simulink library "Crazyflie_Library"  (R2019a)
settings: Solver=VariableStepAuto  StartTime=0.0  StopTime=10.0  RelTol=1e-3
values from neighbouring files (symbols this model uses):
  DeePC_param = evalin('base', 'DeePC_param')    [DeePC_Optimizer_osqp.m]
  param = evalin('base', 'param')    [DeePC_Optimizer_osqp.m]    (also in DeePC_main.m = load_crazyflie_parameters(i_aux))
undefined symbols (not defined in the file or in its folder): DiscIntNeverNeededParam
libraries: simulink x3, $bdroot x3
(part 1 of 2)
settings Model: Creator=ezzat  LastModifiedBy=ezzat
settings DataIOCC: ReturnWorkspaceOutputs=off
settings DebuggingCC: ArithmeticOperatorsInVariantConditions=warning

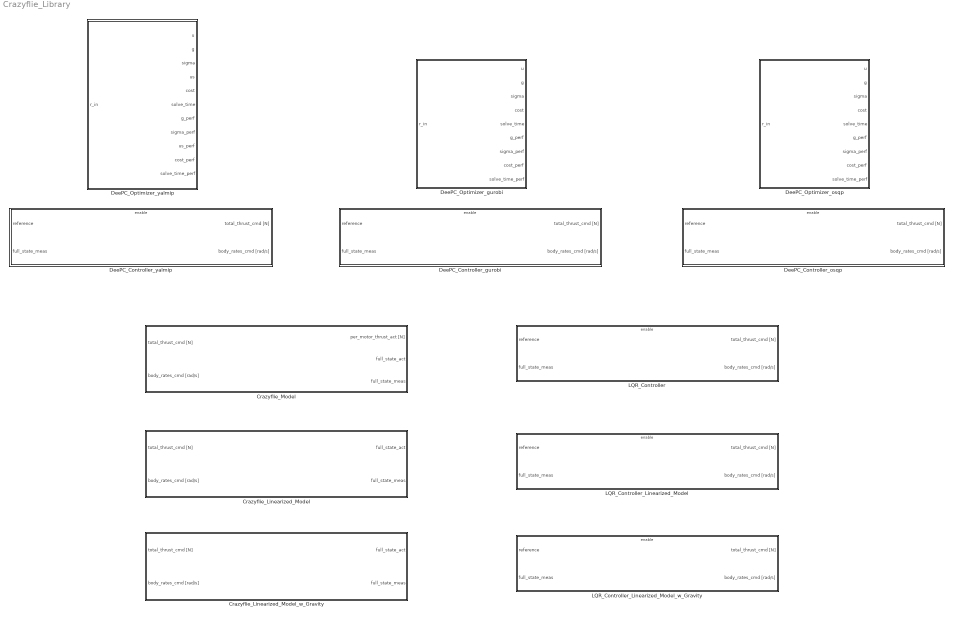
== system Crazyflie_Library ==
  Crazyflie_Linearized_Model : Subsystem
  Crazyflie_Linearized_Model_w_Gravity : Subsystem
  Crazyflie_Model : Subsystem
  DeePC_Controller_gurobi : Subsystem
  DeePC_Controller_osqp : Subsystem
  DeePC_Controller_yalmip : Subsystem
  DeePC_Optimizer_gurobi : Subsystem
  DeePC_Optimizer_osqp : Subsystem
  DeePC_Optimizer_yalmip : Subsystem
  LQR_Controller : Subsystem
  LQR_Controller_Linearized_Model : Subsystem
  LQR_Controller_Linearized_Model_w_Gravity : Subsystem

== system Crazyflie_Library/Crazyflie_Linearized_Model ==
  note: full state measurement
      | (x, y, z, x_dot, y_dot, z_dot, roll, pitch, yaw, roll_dot, pitch_dot, yaw_dot)
  total_thrust_cmd [N] : Inport
  body_rates_cmd [rad/s] : Inport  Port=2
  Add : Sum
  Gain : Gain  Gain=param.Bc  Multiplication=Matrix(K*u)
  Gain1 : Gain  Gain=param.Ac  Multiplication=Matrix(K*u)
  Integrator : Integrator  InitialCondition=param.nrotor_initial_condition(1:9)
  Measurements : Subsystem
  Mux : Mux  Inputs=2
  Mux1 : Mux  Inputs=2
  Unit Delay : UnitDelay  InitialCondition=param.nrotor_initial_condition(10:12)  SampleTime=param.sample_time_controller_inner  HasFrameUpgradeWarning=on
  full_state_act : Outport
  full_state_meas : Outport  Port=2
  wires:
  Measurements/1(full state measurements) -> full_state_meas/1
  total_thrust_cmd [N]/1 -> Mux/1
  body_rates_cmd [rad/s]/1 -> Unit Delay/1, Mux/2
  Mux/1 -> Gain/1
  Gain/1 -> Add/1
  Gain1/1 -> Add/2
  Add/1 -> Integrator/1
  Integrator/1 -> Mux1/1, Gain1/1
  Mux1/1 -> full_state_act/1, Measurements/1(full state)
  Unit Delay/1 -> Mux1/2

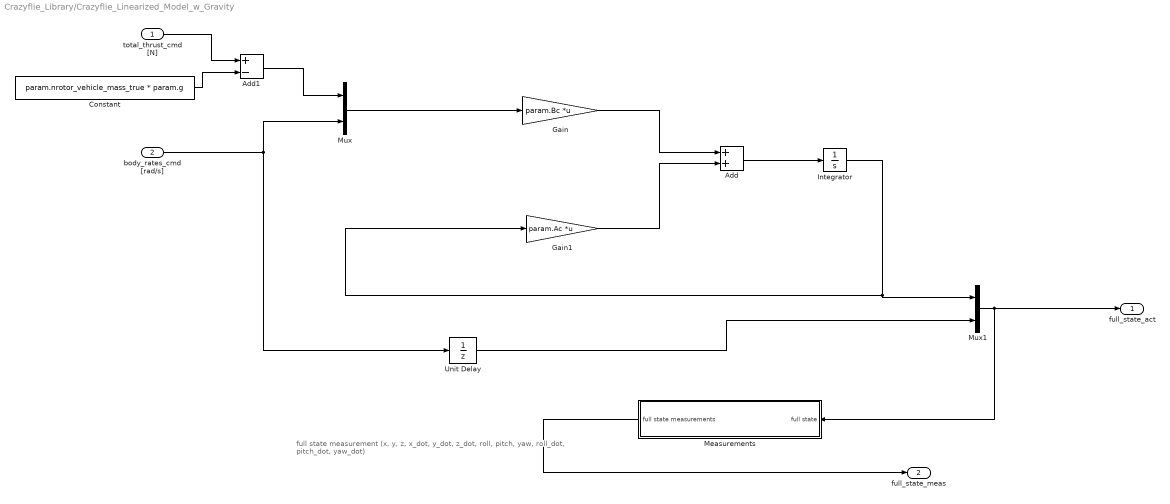
== system Crazyflie_Library/Crazyflie_Linearized_Model_w_Gravity ==
  note: full state measurement
      | (x, y, z, x_dot, y_dot, z_dot, roll, pitch, yaw, roll_dot, pitch_dot, yaw_dot)
  total_thrust_cmd [N] : Inport
  body_rates_cmd [rad/s] : Inport  Port=2
  Add : Sum
  Add1 : Sum  Inputs=+-
  Constant : Constant  Value=param.nrotor_vehicle_mass_true * param.g
  Gain : Gain  Gain=param.Bc  Multiplication=Matrix(K*u)
  Gain1 : Gain  Gain=param.Ac  Multiplication=Matrix(K*u)
  Integrator : Integrator  InitialCondition=param.nrotor_initial_condition(1:9)
  Measurements : Subsystem
  Mux : Mux  Inputs=2
  Mux1 : Mux  Inputs=2
  Unit Delay : UnitDelay  InitialCondition=param.nrotor_initial_condition(10:12)  SampleTime=param.sample_time_controller_inner  HasFrameUpgradeWarning=on
  full_state_act : Outport
  full_state_meas : Outport  Port=2
  wires:
  Measurements/1(full state measurements) -> full_state_meas/1
  body_rates_cmd [rad/s]/1 -> Unit Delay/1, Mux/2
  Mux/1 -> Gain/1
  Gain/1 -> Add/1
  Gain1/1 -> Add/2
  Add/1 -> Integrator/1
  Integrator/1 -> Mux1/1, Gain1/1
  Mux1/1 -> full_state_act/1, Measurements/1(full state)
  total_thrust_cmd [N]/1 -> Add1/1
  Add1/1 -> Mux/1
  Constant/1 -> Add1/2
  Unit Delay/1 -> Mux1/2

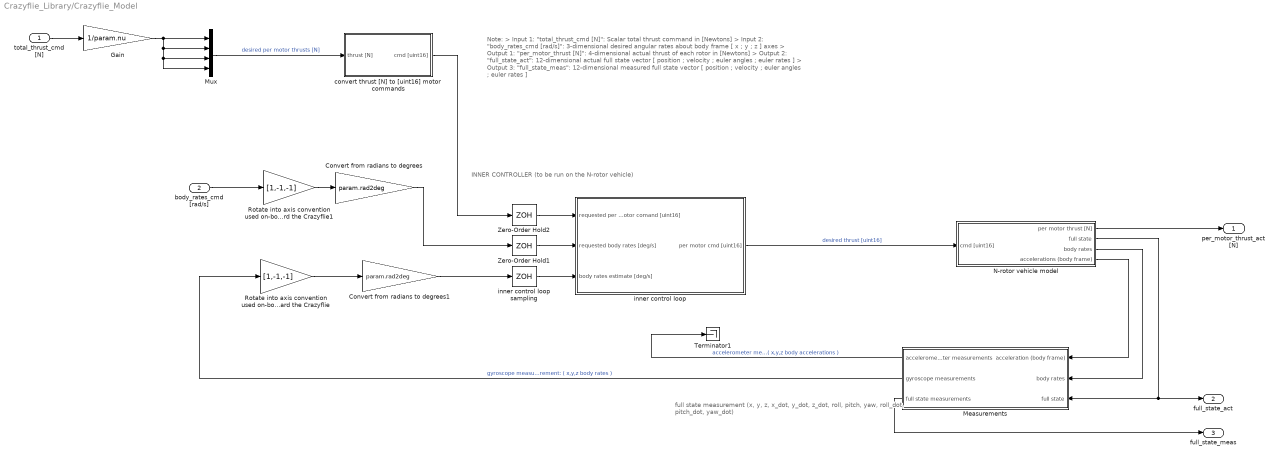
== system Crazyflie_Library/Crazyflie_Model ==
  note: Note:
      | > Input 1: "total_thrust_cmd [N]": Scalar total thrust command in [Newtons]
      | > Input 2: "body_rates_cmd [rad/s]": 3-dimensional desired angular rates about body frame [ x ; y ; z ] axes
      | > Output 1: "per_motor_thrust [N]": 4-dimensional actual thrust of each rotor in [Newtons]
      | > Output 2: "full_state_act": 12-dimensional actual full state vector [ position ; velocity ; euler angles ; euler rates ]
      | > Output 3: "full_state_meas": 12-dimensional measured full state vector [ position ; velocity ; euler angles ; euler rates ]
  note: full state measurement
      | (x, y, z, x_dot, y_dot, z_dot, roll, pitch, yaw, roll_dot, pitch_dot, yaw_dot)
  note: INNER CONTROLLER (to be run on the N-rotor vehicle)
  total_thrust_cmd [N] : Inport
  body_rates_cmd [rad/s] : Inport  Port=2
  Convert from radians to degrees : Gain  Gain=param.rad2deg
  Convert from radians to degrees1 : Gain  Gain=param.rad2deg
  Gain : Gain  Gain=1/param.nu
  Measurements : Subsystem
  Mux : Mux  Inputs=param.nu
  N-rotor vehicle model : Subsystem
  Rotate into axis convention used on-board the Crazyflie1 : Gain  Gain=[1,-1,-1]
  Rotate into axis convention used on-board the Crazyflie : Gain  Gain=[1,-1,-1]
  Terminator1 : Terminator
  Zero-Order Hold1 : ZeroOrderHold  SampleTime=param.sample_time_controller_inner
  Zero-Order Hold2 : ZeroOrderHold  SampleTime=param.sample_time_controller_inner
  convert thrust [N] to [uint16] motor commands : Subsystem
  inner control loop sampling : ZeroOrderHold  SampleTime=param.sample_time_controller_inner
  inner control loop : Subsystem
  "per_motor_thrust_act [N] " : Outport
  full_state_act : Outport  Port=2
  full_state_meas : Outport  Port=3
  wires:
  Gain/1 -> Mux/4, Mux/3, Mux/2, Mux/1
  Zero-Order Hold1/1 -> inner control loop/2(requested body rates [deg/s])
  Convert from radians to degrees/1 -> Zero-Order Hold1/1
  Mux/1 -> convert thrust [N] to [uint16] motor commands/1(thrust [N])  "desired per motor thrusts [N]"
  Measurements/1(accelerometer measurements) -> Terminator1/1  "accelerometer measurement: ( x,y,z body accelerations )"
  N-rotor vehicle model/2(full state) -> Measurements/3(full state), full_state_act/1
  body_rates_cmd [rad/s]/1 -> Rotate into axis convention used on-board the Crazyflie1/1
  N-rotor vehicle model/1(per motor thrust [N]) -> "per_motor_thrust_act [N] "/1
  N-rotor vehicle model/3(body rates) -> Measurements/2(body rates)
  Measurements/3(full state measurements) -> full_state_meas/1
  Convert from radians to degrees1/1 -> inner control loop sampling/1
  inner control loop/1(per motor cmd [uint16]) -> N-rotor vehicle model/1(cmd [uint16])  "desired thrust [uint16]"
  Rotate into axis convention used on-board the Crazyflie/1 -> Convert from radians to degrees1/1
  Zero-Order Hold2/1 -> inner control loop/1(requested per motor comand [uint16])
  N-rotor vehicle model/4(accelerations (body frame)) -> Measurements/1(acceleration (body frame))
  total_thrust_cmd [N]/1 -> Gain/1
  convert thrust [N] to [uint16] motor commands/1(cmd [uint16]) -> Zero-Order Hold2/1
  inner control loop sampling/1 -> inner control loop/3(body rates estimate [deg/s])
  Measurements/2(gyroscope measurements) -> Rotate into axis convention used on-board the Crazyflie/1  "gyroscope measurement: ( x,y,z body rates )"
  Rotate into axis convention used on-board the Crazyflie1/1 -> Convert from radians to degrees/1

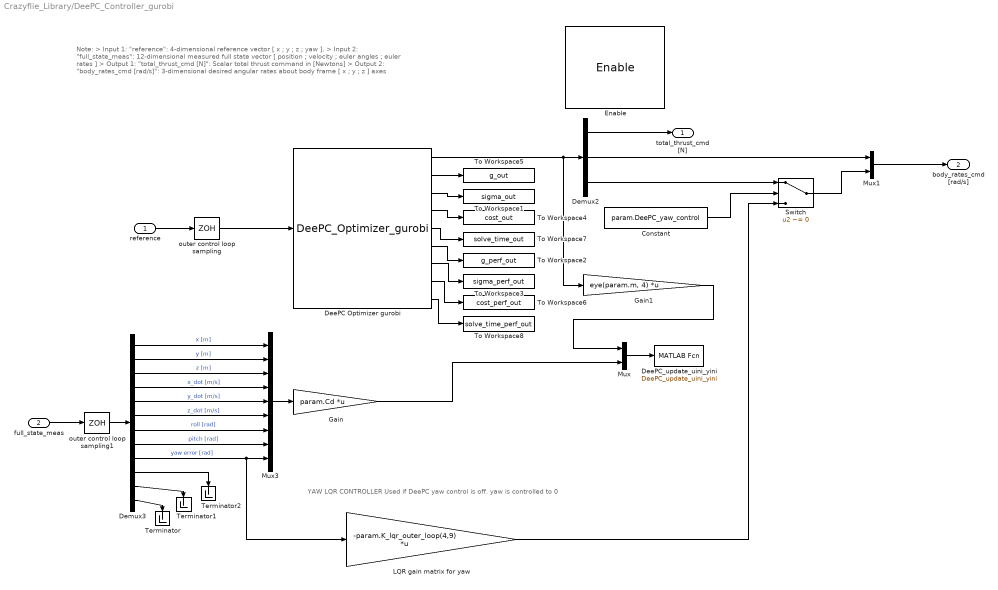
== system Crazyflie_Library/DeePC_Controller_gurobi ==
  note: Note:
      | > Input 1: "reference": 4-dimensional reference vector [ x ; y ; z ; yaw ].
      | > Input 2: "full_state_meas": 12-dimensional measured full state vector [ position ; velocity ; euler angles ; euler rates ]
      | > Output 1: "total_thrust_cmd [N]": Scalar total thrust command in [Newtons]
      | > Output 2: "body_rates_cmd [rad/s]": 3-dimensional desired angular rates about body frame [ x ; y ; z ] axes
  note: YAW LQR CONTROLLER
      | Used if DeePC yaw control is off. yaw is controlled to 0
  reference : Inport
  full_state_meas : Inport  Port=2
  Enable : EnablePort
  Constant : Constant  Value=param.DeePC_yaw_control
  DeePC Optimizer gurobi : $bdroot/DeePC_Optimizer_gurobi  SystemSampleTime=-1
  DeePC_update_uini_yini : MATLABFcn  MATLABFcn=DeePC_update_uini_yini  OutputDimensions=0
  Demux2 : Demux  Outputs=[1 2 1]
  Demux3 : Demux  Outputs=12
  Gain : Gain  Gain=param.Cd  Multiplication=Matrix(K*u)
  Gain1 : Gain  Gain=eye(param.m, 4)  Multiplication=Matrix(K*u)
  LQR gain matrix for yaw : Gain  Gain=-param.K_lqr_outer_loop(4,9)  Multiplication=Matrix(K*u)
  Mux : Mux  Inputs=2
  Mux1 : Mux  Inputs=[2 1]
  Mux3 : Mux  Inputs=9
  Switch : Switch  Criteria=u2 ~= 0
  Terminator : Terminator
  Terminator1 : Terminator
  Terminator2 : Terminator
  To Workspace1 : ToWorkspace  VariableName=sigma_out  SampleTime=-1
  To Workspace2 : ToWorkspace  VariableName=g_perf_out  SampleTime=-1
  To Workspace3 : ToWorkspace  VariableName=sigma_perf_out  SampleTime=-1
  To Workspace4 : ToWorkspace  VariableName=cost_out  SampleTime=-1
  To Workspace5 : ToWorkspace  VariableName=g_out  SampleTime=-1
  To Workspace6 : ToWorkspace  VariableName=cost_perf_out  SampleTime=-1
  To Workspace7 : ToWorkspace  VariableName=solve_time_out  SampleTime=-1
  To Workspace8 : ToWorkspace  VariableName=solve_time_perf_out  SampleTime=-1
  outer control loop sampling : ZeroOrderHold  SampleTime=param.sample_time_controller_outer
  outer control loop sampling1 : ZeroOrderHold  SampleTime=param.sample_time_controller_outer
  total_thrust_cmd [N] : Outport
  body_rates_cmd [rad/s] : Outport  Port=2
  wires:
  Demux3/11 -> Terminator1/1
  Demux3/1 -> Mux3/1  "x [m]"
  Demux3/3 -> Mux3/3  "z [m]"
  Demux3/6 -> Mux3/6  "z_dot [m/s]"
  Demux3/2 -> Mux3/2  "y [m]"
  Demux3/8 -> Mux3/8  "pitch [rad]"
  Demux3/12 -> Terminator/1
  Demux3/7 -> Mux3/7  "roll [rad]"
  Demux3/10 -> Terminator2/1
  Demux3/4 -> Mux3/4  "x_dot [m/s]"
  Demux3/5 -> Mux3/5  "y_dot [m/s]"
  full_state_meas/1 -> outer control loop sampling1/1
  reference/1 -> outer control loop sampling/1
  outer control loop sampling1/1 -> Demux3/1
  Mux3/1 -> Gain/1
  Demux2/1 -> total_thrust_cmd [N]/1
  outer control loop sampling/1 -> DeePC Optimizer gurobi/1
  Mux/1 -> DeePC_update_uini_yini/1
  Gain/1 -> Mux/2
  DeePC Optimizer gurobi/1 -> Gain1/1, Demux2/1
  Demux2/2 -> Mux1/1
  Mux1/1 -> body_rates_cmd [rad/s]/1
  LQR gain matrix for yaw/1 -> Switch/3
  Demux3/9 -> LQR gain matrix for yaw/1, Mux3/9  "yaw error [rad]"
  Demux2/3 -> Switch/1
  Switch/1 -> Mux1/2
  Constant/1 -> Switch/2
  Gain1/1 -> Mux/1
  DeePC Optimizer gurobi/2 -> To Workspace5/1
  DeePC Optimizer gurobi/9 -> To Workspace8/1
  DeePC Optimizer gurobi/5 -> To Workspace7/1
  DeePC Optimizer gurobi/6 -> To Workspace2/1
  DeePC Optimizer gurobi/8 -> To Workspace6/1
  DeePC Optimizer gurobi/3 -> To Workspace1/1
  DeePC Optimizer gurobi/4 -> To Workspace4/1
  DeePC Optimizer gurobi/7 -> To Workspace3/1

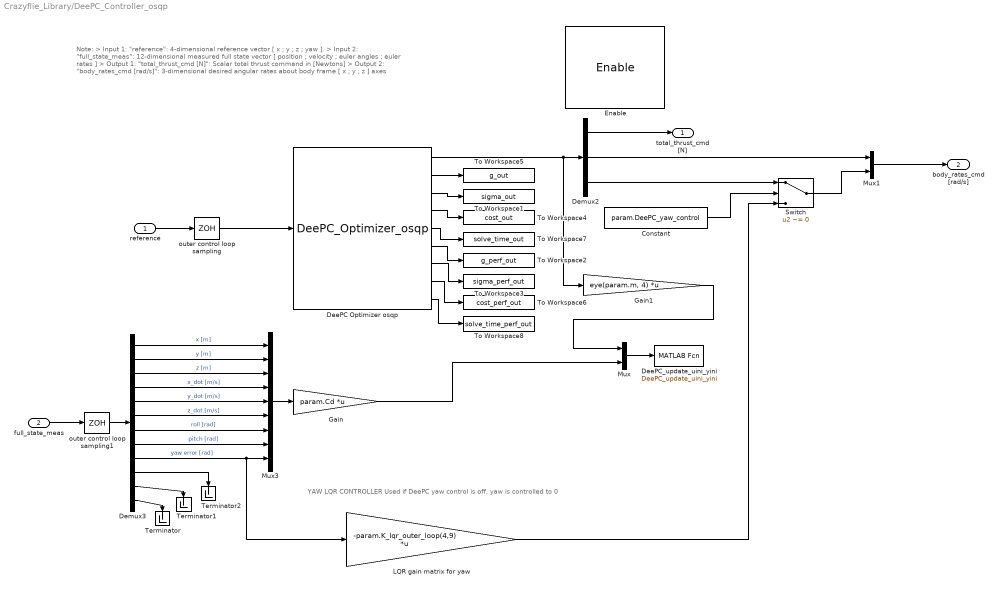
== system Crazyflie_Library/DeePC_Controller_osqp ==
  note: Note:
      | > Input 1: "reference": 4-dimensional reference vector [ x ; y ; z ; yaw ].
      | > Input 2: "full_state_meas": 12-dimensional measured full state vector [ position ; velocity ; euler angles ; euler rates ]
      | > Output 1: "total_thrust_cmd [N]": Scalar total thrust command in [Newtons]
      | > Output 2: "body_rates_cmd [rad/s]": 3-dimensional desired angular rates about body frame [ x ; y ; z ] axes
  note: YAW LQR CONTROLLER
      | Used if DeePC yaw control is off. yaw is controlled to 0
  reference : Inport
  full_state_meas : Inport  Port=2
  Enable : EnablePort
  Constant : Constant  Value=param.DeePC_yaw_control
  DeePC Optimizer osqp : $bdroot/DeePC_Optimizer_osqp  SystemSampleTime=-1
  DeePC_update_uini_yini : MATLABFcn  MATLABFcn=DeePC_update_uini_yini  OutputDimensions=0
  Demux2 : Demux  Outputs=[1 2 1]
  Demux3 : Demux  Outputs=12
  Gain : Gain  Gain=param.Cd  Multiplication=Matrix(K*u)
  Gain1 : Gain  Gain=eye(param.m, 4)  Multiplication=Matrix(K*u)
  LQR gain matrix for yaw : Gain  Gain=-param.K_lqr_outer_loop(4,9)  Multiplication=Matrix(K*u)
  Mux : Mux  Inputs=2
  Mux1 : Mux  Inputs=[2 1]
  Mux3 : Mux  Inputs=9
  Switch : Switch  Criteria=u2 ~= 0
  Terminator : Terminator
  Terminator1 : Terminator
  Terminator2 : Terminator
  To Workspace1 : ToWorkspace  VariableName=sigma_out  SampleTime=-1
  To Workspace2 : ToWorkspace  VariableName=g_perf_out  SampleTime=-1
  To Workspace3 : ToWorkspace  VariableName=sigma_perf_out  SampleTime=-1
  To Workspace4 : ToWorkspace  VariableName=cost_out  SampleTime=-1
  To Workspace5 : ToWorkspace  VariableName=g_out  SampleTime=-1
  To Workspace6 : ToWorkspace  VariableName=cost_perf_out  SampleTime=-1
  To Workspace7 : ToWorkspace  VariableName=solve_time_out  SampleTime=-1
  To Workspace8 : ToWorkspace  VariableName=solve_time_perf_out  SampleTime=-1
  outer control loop sampling : ZeroOrderHold  SampleTime=param.sample_time_controller_outer
  outer control loop sampling1 : ZeroOrderHold  SampleTime=param.sample_time_controller_outer
  total_thrust_cmd [N] : Outport
  body_rates_cmd [rad/s] : Outport  Port=2
  wires:
  Demux3/11 -> Terminator1/1
  Demux3/1 -> Mux3/1  "x [m]"
  Demux3/3 -> Mux3/3  "z [m]"
  Demux3/6 -> Mux3/6  "z_dot [m/s]"
  Demux3/2 -> Mux3/2  "y [m]"
  Demux3/8 -> Mux3/8  "pitch [rad]"
  Demux3/12 -> Terminator/1
  Demux3/7 -> Mux3/7  "roll [rad]"
  Demux3/10 -> Terminator2/1
  Demux3/4 -> Mux3/4  "x_dot [m/s]"
  Demux3/5 -> Mux3/5  "y_dot [m/s]"
  full_state_meas/1 -> outer control loop sampling1/1
  reference/1 -> outer control loop sampling/1
  outer control loop sampling1/1 -> Demux3/1
  Mux3/1 -> Gain/1
  Demux2/1 -> total_thrust_cmd [N]/1
  outer control loop sampling/1 -> DeePC Optimizer osqp/1
  Mux/1 -> DeePC_update_uini_yini/1
  Gain/1 -> Mux/2
  DeePC Optimizer osqp/1 -> Gain1/1, Demux2/1
  Demux2/2 -> Mux1/1
  Mux1/1 -> body_rates_cmd [rad/s]/1
  LQR gain matrix for yaw/1 -> Switch/3
  Demux3/9 -> LQR gain matrix for yaw/1, Mux3/9  "yaw error [rad]"
  Demux2/3 -> Switch/1
  Switch/1 -> Mux1/2
  Constant/1 -> Switch/2
  Gain1/1 -> Mux/1
  DeePC Optimizer osqp/2 -> To Workspace5/1
  DeePC Optimizer osqp/9 -> To Workspace8/1
  DeePC Optimizer osqp/5 -> To Workspace7/1
  DeePC Optimizer osqp/6 -> To Workspace2/1
  DeePC Optimizer osqp/8 -> To Workspace6/1
  DeePC Optimizer osqp/3 -> To Workspace1/1
  DeePC Optimizer osqp/4 -> To Workspace4/1
  DeePC Optimizer osqp/7 -> To Workspace3/1

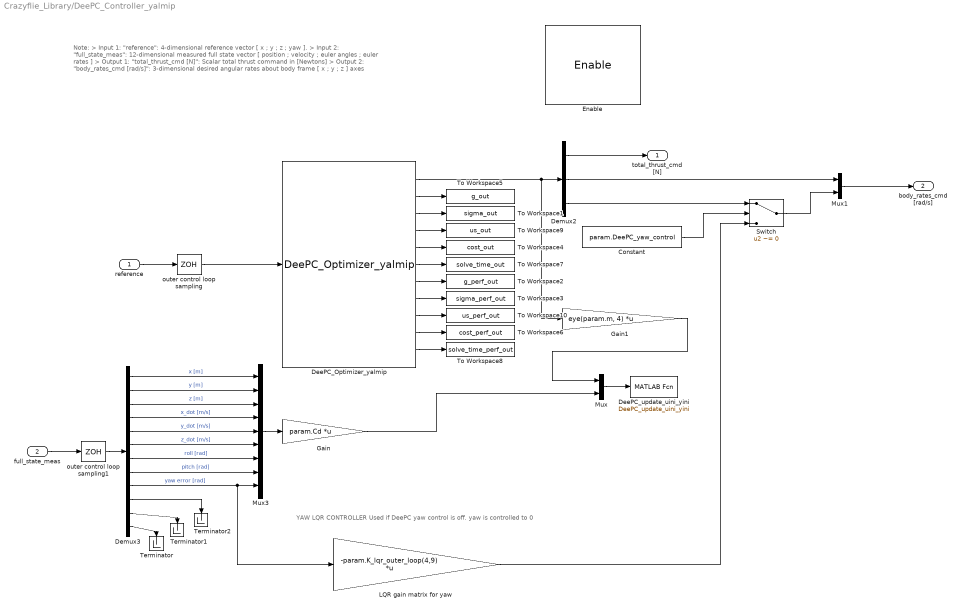
== system Crazyflie_Library/DeePC_Controller_yalmip ==
  note: Note:
      | > Input 1: "reference": 4-dimensional reference vector [ x ; y ; z ; yaw ].
      | > Input 2: "full_state_meas": 12-dimensional measured full state vector [ position ; velocity ; euler angles ; euler rates ]
      | > Output 1: "total_thrust_cmd [N]": Scalar total thrust command in [Newtons]
      | > Output 2: "body_rates_cmd [rad/s]": 3-dimensional desired angular rates about body frame [ x ; y ; z ] axes
  note: YAW LQR CONTROLLER
      | Used if DeePC yaw control is off. yaw is controlled to 0
  reference : Inport
  full_state_meas : Inport  Port=2
  Enable : EnablePort
  Constant : Constant  Value=param.DeePC_yaw_control
  DeePC_Optimizer_yalmip : $bdroot/DeePC_Optimizer_yalmip  SystemSampleTime=-1
  DeePC_update_uini_yini : MATLABFcn  MATLABFcn=DeePC_update_uini_yini  OutputDimensions=0
  Demux2 : Demux  Outputs=[1 2 1]
  Demux3 : Demux  Outputs=12
  Gain : Gain  Gain=param.Cd  Multiplication=Matrix(K*u)
  Gain1 : Gain  Gain=eye(param.m, 4)  Multiplication=Matrix(K*u)
  LQR gain matrix for yaw : Gain  Gain=-param.K_lqr_outer_loop(4,9)  Multiplication=Matrix(K*u)
  Mux : Mux  Inputs=2
  Mux1 : Mux  Inputs=[2 1]
  Mux3 : Mux  Inputs=9
  Switch : Switch  Criteria=u2 ~= 0
  Terminator : Terminator
  Terminator1 : Terminator
  Terminator2 : Terminator
  To Workspace1 : ToWorkspace  VariableName=sigma_out  SampleTime=-1
  To Workspace10 : ToWorkspace  VariableName=us_perf_out  SampleTime=-1
  To Workspace2 : ToWorkspace  VariableName=g_perf_out  SampleTime=-1
  To Workspace3 : ToWorkspace  VariableName=sigma_perf_out  SampleTime=-1
  To Workspace4 : ToWorkspace  VariableName=cost_out  SampleTime=-1
  To Workspace5 : ToWorkspace  VariableName=g_out  SampleTime=-1
  To Workspace6 : ToWorkspace  VariableName=cost_perf_out  SampleTime=-1
  To Workspace7 : ToWorkspace  VariableName=solve_time_out  SampleTime=-1
  To Workspace8 : ToWorkspace  VariableName=solve_time_perf_out  SampleTime=-1
  To Workspace9 : ToWorkspace  VariableName=us_out  SampleTime=-1
  outer control loop sampling : ZeroOrderHold  SampleTime=param.sample_time_controller_outer
  outer control loop sampling1 : ZeroOrderHold  SampleTime=param.sample_time_controller_outer
  total_thrust_cmd [N] : Outport
  body_rates_cmd [rad/s] : Outport  Port=2
  wires:
  Demux3/11 -> Terminator1/1
  Demux3/1 -> Mux3/1  "x [m]"
  Demux3/3 -> Mux3/3  "z [m]"
  Demux3/6 -> Mux3/6  "z_dot [m/s]"
  Demux3/2 -> Mux3/2  "y [m]"
  Demux3/8 -> Mux3/8  "pitch [rad]"
  Demux3/12 -> Terminator/1
  Demux3/7 -> Mux3/7  "roll [rad]"
  Demux3/10 -> Terminator2/1
  Demux3/4 -> Mux3/4  "x_dot [m/s]"
  Demux3/5 -> Mux3/5  "y_dot [m/s]"
  full_state_meas/1 -> outer control loop sampling1/1
  reference/1 -> outer control loop sampling/1
  outer control loop sampling1/1 -> Demux3/1
  Mux3/1 -> Gain/1
  Demux2/1 -> total_thrust_cmd [N]/1
  DeePC_Optimizer_yalmip/2 -> To Workspace5/1
  DeePC_Optimizer_yalmip/3 -> To Workspace1/1
  outer control loop sampling/1 -> DeePC_Optimizer_yalmip/1
  Mux/1 -> DeePC_update_uini_yini/1
  Gain/1 -> Mux/2
  Demux2/2 -> Mux1/1
  Mux1/1 -> body_rates_cmd [rad/s]/1
  LQR gain matrix for yaw/1 -> Switch/3
  Demux3/9 -> LQR gain matrix for yaw/1, Mux3/9  "yaw error [rad]"
  Demux2/3 -> Switch/1
  Switch/1 -> Mux1/2
  Constant/1 -> Switch/2
  Gain1/1 -> Mux/1
  DeePC_Optimizer_yalmip/1 -> Gain1/1, Demux2/1
  DeePC_Optimizer_yalmip/5 -> To Workspace4/1
  DeePC_Optimizer_yalmip/4 -> To Workspace9/1
  DeePC_Optimizer_yalmip/6 -> To Workspace7/1
  DeePC_Optimizer_yalmip/7 -> To Workspace2/1
  DeePC_Optimizer_yalmip/8 -> To Workspace3/1
  DeePC_Optimizer_yalmip/11 -> To Workspace8/1
  DeePC_Optimizer_yalmip/10 -> To Workspace6/1
  DeePC_Optimizer_yalmip/9 -> To Workspace10/1

== system Crazyflie_Library/DeePC_Optimizer_gurobi ==
  r_in : Inport
  DeePC_Optimizer_gurobi : MATLABFcn  MATLABFcn=DeePC_Optimizer_gurobi  OutputDimensions=2 * (DeePC_param.Ng + DeePC_param.Ns + 2) + 4
  Demux : Demux  Outputs=[DeePC_param.Ng DeePC_param.Ns 1 1 DeePC_param.Ng DeePC_param.Ns 1 1 4]
  u : Outport
  g : Outport  Port=2
  sigma : Outport  Port=3
  cost : Outport  Port=4
  solve_time : Outport  Port=5
  g_perf : Outport  Port=6
  sigma_perf : Outport  Port=7
  cost_perf : Outport  Port=8
  solve_time_perf : Outport  Port=9
  wires:
  r_in/1 -> DeePC_Optimizer_gurobi/1
  Demux/8 -> solve_time_perf/1
  Demux/6 -> sigma_perf/1
  Demux/2 -> sigma/1
  Demux/4 -> solve_time/1
  Demux/9 -> u/1
  Demux/5 -> g_perf/1
  Demux/7 -> cost_perf/1
  Demux/1 -> g/1
  DeePC_Optimizer_gurobi/1 -> Demux/1
  Demux/3 -> cost/1

== system Crazyflie_Library/DeePC_Optimizer_osqp ==
  r_in : Inport
  DeePC_Optimizer_osqp : MATLABFcn  MATLABFcn=DeePC_Optimizer_osqp  OutputDimensions=2 * (DeePC_param.Ng + DeePC_param.Ns + 2) + 4
  Demux : Demux  Outputs=[DeePC_param.Ng DeePC_param.Ns 1 1 DeePC_param.Ng DeePC_param.Ns 1 1 4]
  u : Outport
  g : Outport  Port=2
  sigma : Outport  Port=3
  cost : Outport  Port=4
  solve_time : Outport  Port=5
  g_perf : Outport  Port=6
  sigma_perf : Outport  Port=7
  cost_perf : Outport  Port=8
  solve_time_perf : Outport  Port=9
  wires:
  r_in/1 -> DeePC_Optimizer_osqp/1
  Demux/8 -> solve_time_perf/1
  Demux/6 -> sigma_perf/1
  Demux/2 -> sigma/1
  Demux/4 -> solve_time/1
  Demux/9 -> u/1
  Demux/5 -> g_perf/1
  Demux/7 -> cost_perf/1
  Demux/1 -> g/1
  DeePC_Optimizer_osqp/1 -> Demux/1
  Demux/3 -> cost/1

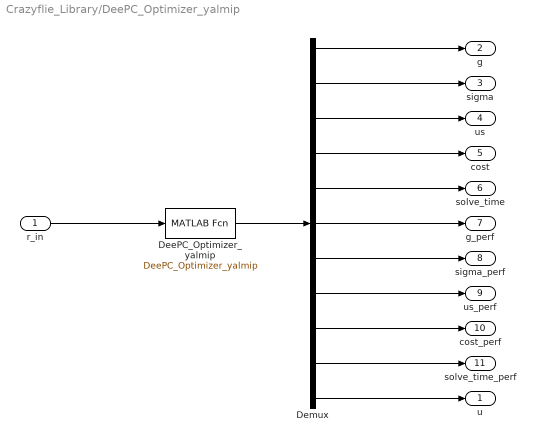
== system Crazyflie_Library/DeePC_Optimizer_yalmip ==
  r_in : Inport
  DeePC_Optimizer_yalmip : MATLABFcn  MATLABFcn=DeePC_Optimizer_yalmip  OutputDimensions=2 * (DeePC_param.Ng + DeePC_param.Ns + param.m + 2) + 4
  Demux : Demux  Outputs=[DeePC_param.Ng DeePC_param.Ns param.m 1 1 DeePC_param.Ng DeePC_param.Ns param.m 1 1 4]
  u : Outport
  g : Outport  Port=2
  sigma : Outport  Port=3
  us : Outport  Port=4
  cost : Outport  Port=5
  solve_time : Outport  Port=6
  g_perf : Outport  Port=7
  sigma_perf : Outport  Port=8
  us_perf : Outport  Port=9
  cost_perf : Outport  Port=10
  solve_time_perf : Outport  Port=11
  wires:
  DeePC_Optimizer_yalmip/1 -> Demux/1
  Demux/1 -> g/1
  Demux/2 -> sigma/1
  r_in/1 -> DeePC_Optimizer_yalmip/1
  Demux/11 -> u/1
  Demux/10 -> solve_time_perf/1
  Demux/9 -> cost_perf/1
  Demux/7 -> sigma_perf/1
  Demux/6 -> g_perf/1
  Demux/5 -> solve_time/1
  Demux/4 -> cost/1
  Demux/3 -> us/1
  Demux/8 -> us_perf/1

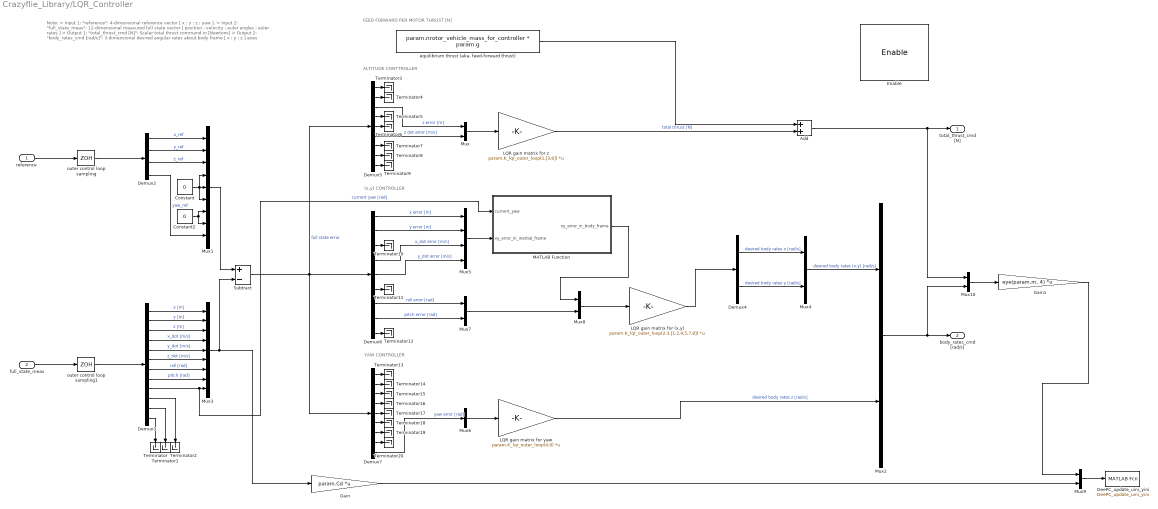
== system Crazyflie_Library/LQR_Controller ==
  note: Note:
      | > Input 1: "reference": 4-dimensional reference vector [ x ; y ; z ; yaw ].
      | > Input 2: "full_state_meas": 12-dimensional measured full state vector [ position ; velocity ; euler angles ; euler rates ]
      | > Output 1: "total_thrust_cmd [N]": Scalar total thrust command in [Newtons]
      | > Output 2: "body_rates_cmd [rad/s]": 3-dimensional desired angular rates about body frame [ x ; y ; z ] axes
  note: ALTITUDE CONTTROLLER
  note: FEED FORWARD PER MOTOR THRUST [N]
  note: YAW CONTROLLER
  note: (x,y) CONTROLLER
  reference : Inport
  full_state_meas : Inport  Port=2
  Enable : EnablePort
  Add : Sum
  Constant : Constant  Value=0
  Constant2 : Constant  Value=0
  DeePC_update_uini_yini : MATLABFcn  MATLABFcn=DeePC_update_uini_yini  OutputDimensions=0
  Demux2 : Demux
  Demux3 : Demux  Outputs=12
  Demux4 : Demux  Outputs=2
  Demux5 : Demux  Outputs=9
  Demux6 : Demux  Outputs=9
  Demux7 : Demux  Outputs=9
  Gain : Gain  Gain=param.Cd  Multiplication=Matrix(K*u)
  Gain1 : Gain  Gain=eye(param.m, 4)  Multiplication=Matrix(K*u)
  LQR gain matrix for (x,y) : Gain  Gain=param.K_lqr_outer_loop(2:3,[1,2,4,5,7,8])  Multiplication=Matrix(K*u)
  LQR gain matrix for yaw : Gain  Gain=param.K_lqr_outer_loop(4,9)  Multiplication=Matrix(K*u)
  LQR gain matrix for z : Gain  Gain=param.K_lqr_outer_loop(1,[3,6])  Multiplication=Matrix(K*u)
  MATLAB Function : MATLAB Function  TreatAsAtomicUnit=on
  Mux{,2,4,7..10} (7 alike) : Mux  Inputs=2
  Mux1 : Mux  Inputs=9
  Mux3 : Mux  Inputs=9
  Mux5 : Mux
  Mux6 : Mux  Inputs=1
  Subtract : Sum  Inputs=+-
  Terminator{,1..20} (21 alike) : Terminator
  equilibrium thrust (aka. feed-forward thrust) : Constant  Value=param.nrotor_vehicle_mass_for_controller * param.g
  outer control loop sampling : ZeroOrderHold  SampleTime=param.sample_time_controller_outer
  outer control loop sampling1 : ZeroOrderHold  SampleTime=param.sample_time_controller_outer
  total_thrust_cmd [N] : Outport
  body_rates_cmd [rad/s] : Outport  Port=2
  wires:
  outer control loop sampling1/1 -> Demux3/1
  reference/1 -> outer control loop sampling/1
  outer control loop sampling/1 -> Demux2/1
  full_state_meas/1 -> outer control loop sampling1/1
  Demux5/1 -> Terminator3/1
  Demux5/5 -> Terminator6/1
  Demux3/5 -> Mux3/5  "y_dot [m/s]"
  Demux4/1 -> Mux4/1  "desired body rates x [rad/s]"
  LQR gain matrix for (x,y)/1 -> Demux4/1
  Demux5/7 -> Terminator7/1
  Mux8/1 -> LQR gain matrix for (x,y)/1
  Mux1/1 -> Subtract/1
  Demux7/7 -> Terminator19/1
  MATLAB Function/1(xy_error_in_body_frame) -> Mux8/1
  Demux6/1 -> Mux5/1  "x error [m]"
  Demux5/2 -> Terminator4/1
  Mux6/1 -> LQR gain matrix for yaw/1
  Demux6/3 -> Terminator10/1
  Demux5/9 -> Terminator9/1
  Mux5/1 -> MATLAB Function/2(xy_error_in_inertial_frame)
  Demux7/8 -> Terminator20/1
  Demux5/3 -> Mux/1  "z error [m]"
  Demux7/1 -> Terminator13/1
  Demux6/7 -> Mux7/1  "roll error [rad]"
  Mux/1 -> LQR gain matrix for z/1
  Demux2/3 -> Mux1/3  "z_ref"
  Demux3/4 -> Mux3/4  "x_dot [m/s]"
  Demux6/8 -> Mux7/2  "pitch error [rad]"
  Demux6/2 -> Mux5/2  "y error [m]"
  Demux5/8 -> Terminator8/1
  Demux6/9 -> Terminator12/1
  Demux7/2 -> Terminator14/1
  LQR gain matrix for yaw/1 -> Mux2/2  "desired body rates z [rad/s]"
  Demux4/2 -> Mux4/2  "desired body rates y [rad/s]"
  Subtract/1 -> Demux7/1, Demux5/1, Demux6/1  "full state error"
  Demux3/10 -> Terminator2/1
  Demux5/6 -> Mux/2  "z dot error [m/s]"
  Demux2/2 -> Mux1/2  "y_ref"
  Demux3/7 -> Mux3/7  "roll [rad]"
  Demux3/9 -> MATLAB Function/1(current_yaw), Mux3/9  "current yaw [rad]"
  Demux3/12 -> Terminator/1
  Demux6/4 -> Mux5/3  "x_dot error [m/s]"
  Demux3/8 -> Mux3/8  "pitch [rad]"
  Demux2/4 -> Mux1/9  "yaw_ref"
  Demux3/2 -> Mux3/2  "y [m]"
  Demux6/6 -> Terminator11/1
  Constant2/1 -> Mux1/8, Mux1/7
  Constant/1 -> Mux1/6, Mux1/4, Mux1/5
  Demux6/5 -> Mux5/4  "y_dot error [m/s]"
  Demux3/6 -> Mux3/6  "z_dot [m/s]"
  Demux3/3 -> Mux3/3  "z [m]"
  Mux4/1 -> Mux2/1  "desired body rates (x,y) [rad/s]"
  Demux7/3 -> Terminator15/1
  Demux3/1 -> Mux3/1  "x [m]"
  Mux7/1 -> Mux8/2
  Demux2/1 -> Mux1/1  "x_ref"
  Demux7/6 -> Terminator18/1
  Demux7/5 -> Terminator17/1
  LQR gain matrix for z/1 -> Add/2  "total thrust [N]"
  Demux7/9 -> Mux6/1  "yaw error [rad]"
  Demux3/11 -> Terminator1/1
  Demux5/4 -> Terminator5/1
  Demux7/4 -> Terminator16/1
  equilibrium thrust (aka. feed-forward thrust)/1 -> Add/1
  Mux9/1 -> DeePC_update_uini_yini/1
  Add/1 -> total_thrust_cmd [N]/1, Mux10/1
  Mux2/1 -> Mux10/2, body_rates_cmd [rad/s]/1
  Mux3/1 -> Gain/1, Subtract/2
  Gain/1 -> Mux9/2
  Gain1/1 -> Mux9/1
  Mux10/1 -> Gain1/1

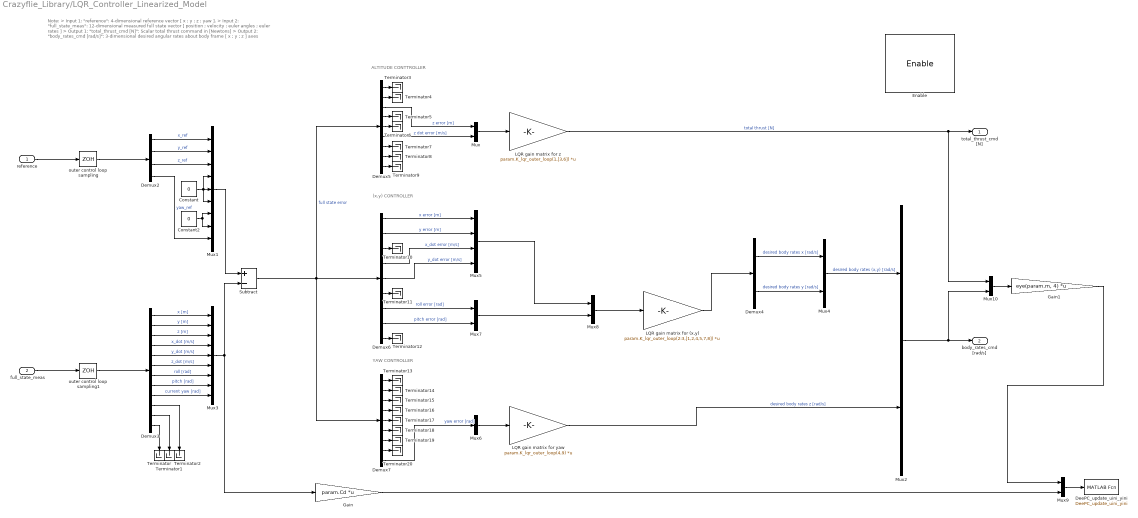
== system Crazyflie_Library/LQR_Controller_Linearized_Model ==
  note: Note:
      | > Input 1: "reference": 4-dimensional reference vector [ x ; y ; z ; yaw ].
      | > Input 2: "full_state_meas": 12-dimensional measured full state vector [ position ; velocity ; euler angles ; euler rates ]
      | > Output 1: "total_thrust_cmd [N]": Scalar total thrust command in [Newtons]
      | > Output 2: "body_rates_cmd [rad/s]": 3-dimensional desired angular rates about body frame [ x ; y ; z ] axes
  note: ALTITUDE CONTTROLLER
  note: YAW CONTROLLER
  note: (x,y) CONTROLLER
  reference : Inport
  full_state_meas : Inport  Port=2
  Enable : EnablePort
  Constant : Constant  Value=0
  Constant2 : Constant  Value=0
  DeePC_update_uini_yini : MATLABFcn  MATLABFcn=DeePC_update_uini_yini  OutputDimensions=0
  Demux2 : Demux
  Demux3 : Demux  Outputs=12
  Demux4 : Demux  Outputs=2
  Demux5 : Demux  Outputs=9
  Demux6 : Demux  Outputs=9
  Demux7 : Demux  Outputs=9
  Gain : Gain  Gain=param.Cd  Multiplication=Matrix(K*u)
  Gain1 : Gain  Gain=eye(param.m, 4)  Multiplication=Matrix(K*u)
  LQR gain matrix for (x,y) : Gain  Gain=param.K_lqr_outer_loop(2:3,[1,2,4,5,7,8])  Multiplication=Matrix(K*u)
  LQR gain matrix for yaw : Gain  Gain=param.K_lqr_outer_loop(4,9)  Multiplication=Matrix(K*u)
  LQR gain matrix for z : Gain  Gain=param.K_lqr_outer_loop(1,[3,6])  Multiplication=Matrix(K*u)
  Mux{,2,4,7..10} (7 alike) : Mux  Inputs=2
  Mux1 : Mux  Inputs=9
  Mux3 : Mux  Inputs=9
  Mux5 : Mux
  Mux6 : Mux  Inputs=1
  Subtract : Sum  Inputs=+-
  Terminator{,1..20} (21 alike) : Terminator
  outer control loop sampling : ZeroOrderHold  SampleTime=param.sample_time_controller_outer
  outer control loop sampling1 : ZeroOrderHold  SampleTime=param.sample_time_controller_outer
  total_thrust_cmd [N] : Outport
  body_rates_cmd [rad/s] : Outport  Port=2
  wires:
  outer control loop sampling1/1 -> Demux3/1
  reference/1 -> outer control loop sampling/1
  outer control loop sampling/1 -> Demux2/1
  full_state_meas/1 -> outer control loop sampling1/1
  Demux5/1 -> Terminator3/1
  Demux5/5 -> Terminator6/1
  Demux3/5 -> Mux3/5  "y_dot [m/s]"
  Demux4/1 -> Mux4/1  "desired body rates x [rad/s]"
  LQR gain matrix for (x,y)/1 -> Demux4/1
  Demux5/7 -> Terminator7/1
  Mux8/1 -> LQR gain matrix for (x,y)/1
  Mux1/1 -> Subtract/1
  Demux7/7 -> Terminator19/1
  Mux5/1 -> Mux8/1
  Demux6/1 -> Mux5/1  "x error [m]"
  Demux5/2 -> Terminator4/1
  Mux6/1 -> LQR gain matrix for yaw/1
  Demux6/3 -> Terminator10/1
  Demux5/9 -> Terminator9/1
  Demux7/8 -> Terminator20/1
  Demux5/3 -> Mux/1  "z error [m]"
  Demux7/1 -> Terminator13/1
  Demux6/7 -> Mux7/1  "roll error [rad]"
  Mux/1 -> LQR gain matrix for z/1
  Demux2/3 -> Mux1/3  "z_ref"
  Demux3/4 -> Mux3/4  "x_dot [m/s]"
  Demux6/8 -> Mux7/2  "pitch error [rad]"
  Demux6/2 -> Mux5/2  "y error [m]"
  Demux5/8 -> Terminator8/1
  Demux6/9 -> Terminator12/1
  Demux7/2 -> Terminator14/1
  LQR gain matrix for yaw/1 -> Mux2/2  "desired body rates z [rad/s]"
  Demux4/2 -> Mux4/2  "desired body rates y [rad/s]"
  Subtract/1 -> Demux7/1, Demux5/1, Demux6/1  "full state error"
  Demux3/10 -> Terminator2/1
  Demux5/6 -> Mux/2  "z dot error [m/s]"
  Demux2/2 -> Mux1/2  "y_ref"
  Demux3/7 -> Mux3/7  "roll [rad]"
  Demux3/9 -> Mux3/9  "current yaw [rad]"
  Demux3/12 -> Terminator/1
  Demux6/4 -> Mux5/3  "x_dot error [m/s]"
  Demux3/8 -> Mux3/8  "pitch [rad]"
  Demux2/4 -> Mux1/9  "yaw_ref"
  Demux3/2 -> Mux3/2  "y [m]"
  Demux6/6 -> Terminator11/1
  Constant2/1 -> Mux1/8, Mux1/7
  Constant/1 -> Mux1/6, Mux1/4, Mux1/5
  Demux6/5 -> Mux5/4  "y_dot error [m/s]"
  Demux3/6 -> Mux3/6  "z_dot [m/s]"
  Demux3/3 -> Mux3/3  "z [m]"
  Mux4/1 -> Mux2/1  "desired body rates (x,y) [rad/s]"
  Demux7/3 -> Terminator15/1
  Demux3/1 -> Mux3/1  "x [m]"
  Mux7/1 -> Mux8/2
  Demux2/1 -> Mux1/1  "x_ref"
  Demux7/6 -> Terminator18/1
  Demux7/5 -> Terminator17/1
  LQR gain matrix for z/1 -> Mux10/1, total_thrust_cmd [N]/1  "total thrust [N]"
  Demux7/9 -> Mux6/1  "yaw error [rad]"
  Demux3/11 -> Terminator1/1
  Demux5/4 -> Terminator5/1
  Demux7/4 -> Terminator16/1
  Mux9/1 -> DeePC_update_uini_yini/1
  Mux2/1 -> Mux10/2, body_rates_cmd [rad/s]/1
  Mux3/1 -> Subtract/2, Gain/1
  Gain/1 -> Mux9/2
  Mux10/1 -> Gain1/1
  Gain1/1 -> Mux9/1

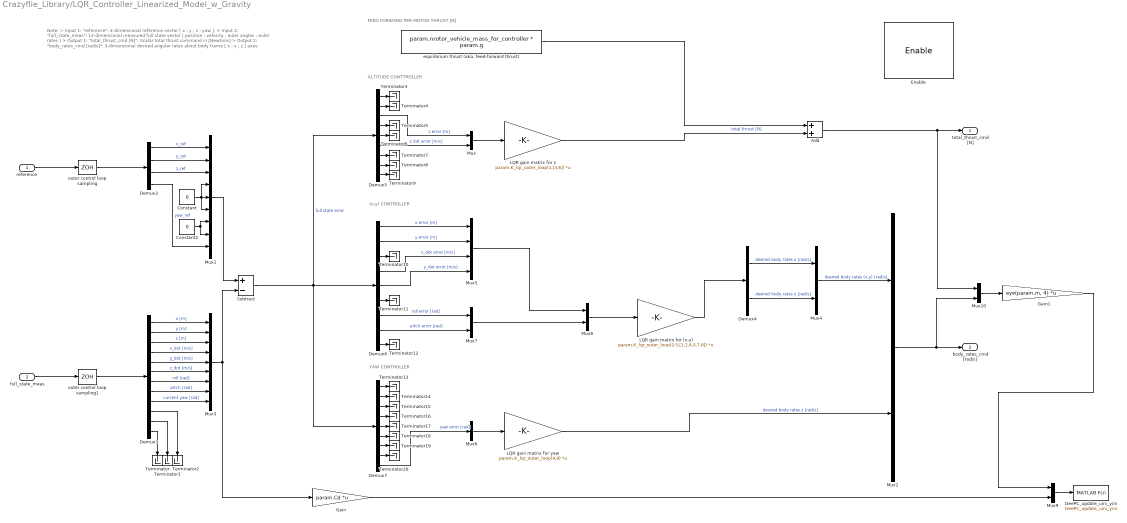
== system Crazyflie_Library/LQR_Controller_Linearized_Model_w_Gravity ==
  note: Note:
      | > Input 1: "reference": 4-dimensional reference vector [ x ; y ; z ; yaw ].
      | > Input 2: "full_state_meas": 12-dimensional measured full state vector [ position ; velocity ; euler angles ; euler rates ]
      | > Output 1: "total_thrust_cmd [N]": Scalar total thrust command in [Newtons]
      | > Output 2: "body_rates_cmd [rad/s]": 3-dimensional desired angular rates about body frame [ x ; y ; z ] axes
  note: ALTITUDE CONTTROLLER
  note: YAW CONTROLLER
  note: (x,y) CONTROLLER
  note: FEED FORWARD PER MOTOR THRUST [N]
  reference : Inport
  full_state_meas : Inport  Port=2
  Enable : EnablePort
  Add : Sum
  Constant : Constant  Value=0
  Constant2 : Constant  Value=0
  DeePC_update_uini_yini : MATLABFcn  MATLABFcn=DeePC_update_uini_yini  OutputDimensions=0
  Demux2 : Demux
  Demux3 : Demux  Outputs=12
  Demux4 : Demux  Outputs=2
  Demux5 : Demux  Outputs=9
  Demux6 : Demux  Outputs=9
  Demux7 : Demux  Outputs=9
  Gain : Gain  Gain=param.Cd  Multiplication=Matrix(K*u)
  Gain1 : Gain  Gain=eye(param.m, 4)  Multiplication=Matrix(K*u)
  LQR gain matrix for (x,y) : Gain  Gain=param.K_lqr_outer_loop(2:3,[1,2,4,5,7,8])  Multiplication=Matrix(K*u)
  LQR gain matrix for yaw : Gain  Gain=param.K_lqr_outer_loop(4,9)  Multiplication=Matrix(K*u)
  LQR gain matrix for z : Gain  Gain=param.K_lqr_outer_loop(1,[3,6])  Multiplication=Matrix(K*u)
  Mux{,2,4,7..10} (7 alike) : Mux  Inputs=2
  Mux1 : Mux  Inputs=9
  Mux3 : Mux  Inputs=9
  Mux5 : Mux
  Mux6 : Mux  Inputs=1
  Subtract : Sum  Inputs=+-
  Terminator{,1..20} (21 alike) : Terminator
  equilibrium thrust (aka. feed-forward thrust) : Constant  Value=param.nrotor_vehicle_mass_for_controller * param.g
  outer control loop sampling : ZeroOrderHold  SampleTime=param.sample_time_controller_outer
  outer control loop sampling1 : ZeroOrderHold  SampleTime=param.sample_time_controller_outer
  total_thrust_cmd [N] : Outport
  body_rates_cmd [rad/s] : Outport  Port=2
  wires:
  Mux2/1 -> Mux10/2, body_rates_cmd [rad/s]/1
  outer control loop sampling1/1 -> Demux3/1
  reference/1 -> outer control loop sampling/1
  outer control loop sampling/1 -> Demux2/1
  full_state_meas/1 -> outer control loop sampling1/1
  Demux5/1 -> Terminator3/1
  Demux5/5 -> Terminator6/1
  Demux3/5 -> Mux3/5  "y_dot [m/s]"
  Demux4/1 -> Mux4/1  "desired body rates x [rad/s]"
  LQR gain matrix for (x,y)/1 -> Demux4/1
  Demux5/7 -> Terminator7/1
  Mux8/1 -> LQR gain matrix for (x,y)/1
  Mux1/1 -> Subtract/1
  Demux7/7 -> Terminator19/1
  Mux5/1 -> Mux8/1
  Demux6/1 -> Mux5/1  "x error [m]"
  Demux5/2 -> Terminator4/1
  Mux6/1 -> LQR gain matrix for yaw/1
  Demux6/3 -> Terminator10/1
  Demux5/9 -> Terminator9/1
  Demux7/8 -> Terminator20/1
  Demux5/3 -> Mux/1  "z error [m]"
  Demux7/1 -> Terminator13/1
  Demux6/7 -> Mux7/1  "roll error [rad]"
  Mux/1 -> LQR gain matrix for z/1
  Demux2/3 -> Mux1/3  "z_ref"
  Demux3/4 -> Mux3/4  "x_dot [m/s]"
  Demux6/8 -> Mux7/2  "pitch error [rad]"
  Demux6/2 -> Mux5/2  "y error [m]"
  Demux5/8 -> Terminator8/1
  Demux6/9 -> Terminator12/1
  Demux7/2 -> Terminator14/1
  LQR gain matrix for yaw/1 -> Mux2/2  "desired body rates z [rad/s]"
  Demux4/2 -> Mux4/2  "desired body rates y [rad/s]"
  Subtract/1 -> Demux7/1, Demux5/1, Demux6/1  "full state error"
  Demux3/10 -> Terminator2/1
  Demux5/6 -> Mux/2  "z dot error [m/s]"
  Demux2/2 -> Mux1/2  "y_ref"
  Demux3/7 -> Mux3/7  "roll [rad]"
  Demux3/9 -> Mux3/9  "current yaw [rad]"
  Demux3/12 -> Terminator/1
  Demux6/4 -> Mux5/3  "x_dot error [m/s]"
  Demux3/8 -> Mux3/8  "pitch [rad]"
  Demux2/4 -> Mux1/9  "yaw_ref"
  Demux3/2 -> Mux3/2  "y [m]"
  Demux6/6 -> Terminator11/1
  Constant2/1 -> Mux1/8, Mux1/7
  Constant/1 -> Mux1/6, Mux1/4, Mux1/5
  Demux6/5 -> Mux5/4  "y_dot error [m/s]"
  Demux3/6 -> Mux3/6  "z_dot [m/s]"
  Demux3/3 -> Mux3/3  "z [m]"
  Mux4/1 -> Mux2/1  "desired body rates (x,y) [rad/s]"
  Demux7/3 -> Terminator15/1
  Demux3/1 -> Mux3/1  "x [m]"
  Mux7/1 -> Mux8/2
  Demux2/1 -> Mux1/1  "x_ref"
  Demux7/6 -> Terminator18/1
  Demux7/5 -> Terminator17/1
  Demux7/9 -> Mux6/1  "yaw error [rad]"
  Demux3/11 -> Terminator1/1
  Demux5/4 -> Terminator5/1
  Demux7/4 -> Terminator16/1
  equilibrium thrust (aka. feed-forward thrust)/1 -> Add/1
  LQR gain matrix for z/1 -> Add/2  "total thrust [N]"
  Add/1 -> Mux10/1, total_thrust_cmd [N]/1
  Mux3/1 -> Gain/1, Subtract/2
  Mux9/1 -> DeePC_update_uini_yini/1
  Gain/1 -> Mux9/2
  Mux10/1 -> Gain1/1
  Gain1/1 -> Mux9/1

== system Crazyflie_Library/Crazyflie_Linearized_Model/Measurements ==
  full state : Inport
  "\"square root\" of the full state covariance matrix" : Constant  Value=param.measurement_noise_full_state_covariance_decomposition
  Add2 : Sum
  draw sample from multivariate Gaussian for full state : MATLAB Function  TreatAsAtomicUnit=on
  full state noise inclusion : Gain  Gain=param.measurement_noise_full_state
  mean vector for the full state : Constant  Value=param.measurement_noise_full_state_mean
  measurement sampling > for Vicon : ZeroOrderHold  SampleTime=param.sample_time_measurements_full_state
  standard normal rand for full state : RandomNumber  Mean=zeros(size(param.measurement_noise_full_state_mean))  Variance=ones(size(param.measurement_noise_full_state_mean))  Seed=param.measurement_noise_full_state_seed  SampleTime=param.sample_time_measurements_full_state  VectorParams1D=off
  full state measurements : Outport
  wires:
  full state/1 -> measurement sampling > for Vicon/1
  measurement sampling > for Vicon/1 -> Add2/2
  "\"square root\" of the full state covariance matrix"/1 -> draw sample from multivariate Gaussian for full state/3(covariance_matrix_decomposition)
  mean vector for the full state/1 -> draw sample from multivariate Gaussian for full state/2(mean_vector)
  standard normal rand for full state/1 -> draw sample from multivariate Gaussian for full state/1(std_normal_rand_sample)
  draw sample from multivariate Gaussian for full state/1(rand_sample) -> full state noise inclusion/1
  full state noise inclusion/1 -> Add2/1
  Add2/1 -> full state measurements/1

== system Crazyflie_Library/Crazyflie_Linearized_Model_w_Gravity/Measurements ==
  full state : Inport
  "\"square root\" of the full state covariance matrix" : Constant  Value=param.measurement_noise_full_state_covariance_decomposition
  Add2 : Sum
  draw sample from multivariate Gaussian for full state : MATLAB Function  TreatAsAtomicUnit=on
  full state noise inclusion : Gain  Gain=param.measurement_noise_full_state
  mean vector for the full state : Constant  Value=param.measurement_noise_full_state_mean
  measurement sampling > for Vicon : ZeroOrderHold  SampleTime=param.sample_time_measurements_full_state
  standard normal rand for full state : RandomNumber  Mean=zeros(size(param.measurement_noise_full_state_mean))  Variance=ones(size(param.measurement_noise_full_state_mean))  Seed=param.measurement_noise_full_state_seed  SampleTime=param.sample_time_measurements_full_state  VectorParams1D=off
  full state measurements : Outport
  wires:
  full state/1 -> measurement sampling > for Vicon/1
  measurement sampling > for Vicon/1 -> Add2/2
  "\"square root\" of the full state covariance matrix"/1 -> draw sample from multivariate Gaussian for full state/3(covariance_matrix_decomposition)
  mean vector for the full state/1 -> draw sample from multivariate Gaussian for full state/2(mean_vector)
  standard normal rand for full state/1 -> draw sample from multivariate Gaussian for full state/1(std_normal_rand_sample)
  draw sample from multivariate Gaussian for full state/1(rand_sample) -> full state noise inclusion/1
  full state noise inclusion/1 -> Add2/1
  Add2/1 -> full state measurements/1

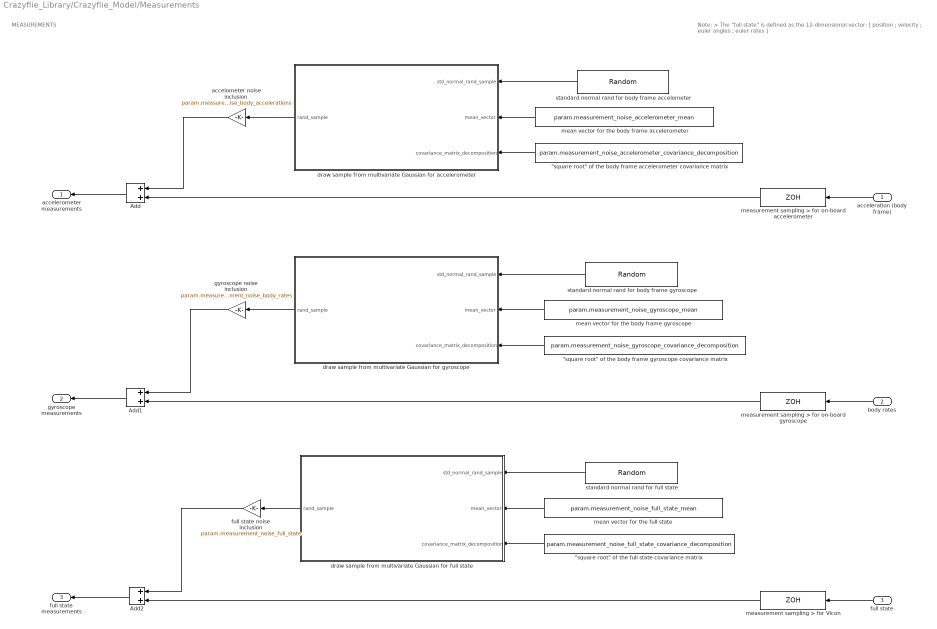
== system Crazyflie_Library/Crazyflie_Model/Measurements ==
  note: Note:
      | > The "full state" is defined as the 12-dimensional vector:
      | [ position ; velocity ; euler angles ; euler rates ]
  note: MEASUREMENTS
  acceleration (body frame) : Inport
  body rates : Inport  Port=2
  full state : Inport  Port=3
  "\"square root\" of the body frame accelerometer covariance matrix" : Constant  Value=param.measurement_noise_accelerometer_covariance_decomposition
  "\"square root\" of the body frame gyroscope covariance matrix" : Constant  Value=param.measurement_noise_gyroscope_covariance_decomposition
  "\"square root\" of the full state covariance matrix" : Constant  Value=param.measurement_noise_full_state_covariance_decomposition
  Add : Sum
  Add1 : Sum
  Add2 : Sum
  accelometer noise inclusion : Gain  Gain=param.measurement_noise_body_accelerations
  draw sample from multivariate Gaussian for accelerometer : MATLAB Function  TreatAsAtomicUnit=on
  draw sample from multivariate Gaussian for full state : MATLAB Function  TreatAsAtomicUnit=on
  draw sample from multivariate Gaussian for gyroscope : MATLAB Function  TreatAsAtomicUnit=on
  full state noise inclusion : Gain  Gain=param.measurement_noise_full_state
  gyroscope noise inclusion : Gain  Gain=param.measurement_noise_body_rates
  mean vector for the body frame accelerometer : Constant  Value=param.measurement_noise_accelerometer_mean
  mean vector for the body frame gyroscope : Constant  Value=param.measurement_noise_gyroscope_mean
  mean vector for the full state : Constant  Value=param.measurement_noise_full_state_mean
  measurement sampling > for Vicon : ZeroOrderHold  SampleTime=param.sample_time_measurements_full_state
  measurement sampling > for on-board accelerometer : ZeroOrderHold  SampleTime=param.sample_time_measurements_body_accelerations
  measurement sampling > for on-board gyroscope : ZeroOrderHold  SampleTime=param.sample_time_measurements_body_rates
  standard normal rand for body frame accelometer : RandomNumber  Mean=zeros(size(param.measurement_noise_accelerometer_mean))  Variance=ones(size(param.measurement_noise_accelerometer_mean))  Seed=param.measurement_noise_accelerometer_seed  SampleTime=param.sample_time_measurements_body_accelerations  VectorParams1D=off
  standard normal rand for body frame gyroscope : RandomNumber  Mean=zeros(size(param.measurement_noise_gyroscope_mean))  Variance=ones(size(param.measurement_noise_gyroscope_mean))  Seed=param.measurement_noise_gyroscope_seed  SampleTime=param.sample_time_measurements_body_rates  VectorParams1D=off
  standard normal rand for full state : RandomNumber  Mean=zeros(size(param.measurement_noise_full_state_mean))  Variance=ones(size(param.measurement_noise_full_state_mean))  Seed=param.measurement_noise_full_state_seed  SampleTime=param.sample_time_measurements_full_state  VectorParams1D=off
  accelerometer measurements : Outport
  gyroscope measurements : Outport  Port=2
  full state measurements : Outport  Port=3
  wires:
  full state/1 -> measurement sampling > for Vicon/1
  acceleration (body frame)/1 -> measurement sampling > for on-board accelerometer/1
  body rates/1 -> measurement sampling > for on-board gyroscope/1
  measurement sampling > for Vicon/1 -> Add2/2
  "\"square root\" of the full state covariance matrix"/1 -> draw sample from multivariate Gaussian for full state/3(covariance_matrix_decomposition)
  mean vector for the full state/1 -> draw sample from multivariate Gaussian for full state/2(mean_vector)
  mean vector for the body frame gyroscope/1 -> draw sample from multivariate Gaussian for gyroscope/2(mean_vector)
  gyroscope noise inclusion/1 -> Add1/1
  measurement sampling > for on-board accelerometer/1 -> Add/2
  mean vector for the body frame accelerometer/1 -> draw sample from multivariate Gaussian for accelerometer/2(mean_vector)
  draw sample from multivariate Gaussian for accelerometer/1(rand_sample) -> accelometer noise inclusion/1
  draw sample from multivariate Gaussian for gyroscope/1(rand_sample) -> gyroscope noise inclusion/1
  standard normal rand for full state/1 -> draw sample from multivariate Gaussian for full state/1(std_normal_rand_sample)
  "\"square root\" of the body frame gyroscope covariance matrix"/1 -> draw sample from multivariate Gaussian for gyroscope/3(covariance_matrix_decomposition)
  accelometer noise inclusion/1 -> Add/1
  draw sample from multivariate Gaussian for full state/1(rand_sample) -> full state noise inclusion/1
  full state noise inclusion/1 -> Add2/1
  measurement sampling > for on-board gyroscope/1 -> Add1/2
  standard normal rand for body frame gyroscope/1 -> draw sample from multivariate Gaussian for gyroscope/1(std_normal_rand_sample)
  standard normal rand for body frame accelometer/1 -> draw sample from multivariate Gaussian for accelerometer/1(std_normal_rand_sample)
  Add2/1 -> full state measurements/1
  "\"square root\" of the body frame accelerometer covariance matrix"/1 -> draw sample from multivariate Gaussian for accelerometer/3(covariance_matrix_decomposition)
  Add/1 -> accelerometer measurements/1
  Add1/1 -> gyroscope measurements/1

== system Crazyflie_Library/Crazyflie_Model/N-rotor vehicle model ==
  note: Note:
      | > The "full state" is defined as the 12-dimensional vector:
      | [ position ; velocity ; euler angles ; euler rates ]
      | > The "thrust [N]" input should be a column vector with
      | length equal to the number of propellers on the vehicle,
      | i.e., with length equal to N
  note: EQUATIONS OF MOTION FOR THE N-ROTOR VEHICLE
  cmd [uint16] : Inport
  DC motor low pass filter{,1..3} (4 alike) : TransferFcn  Denominator=[param.nrotor_tau_M 1]
  Demux : Demux
  Full equations of motions implemented in one shot : Subsystem
  Mux : Mux
  convert motor comand to thrust : Subsystem
  ensure data type is unit16 : DataTypeConversion  OutDataTypeStr=uint16
  per motor thrust [N] : Outport
  full state : Outport  Port=2
  body rates : Outport  Port=3
  accelerations (body frame) : Outport  Port=4
  wires:
  cmd [uint16]/1 -> ensure data type is unit16/1
  Full equations of motions implemented in one shot/1(full state) -> full state/1
  Full equations of motions implemented in one shot/2(body rates) -> body rates/1
  Full equations of motions implemented in one shot/3(body accellerations) -> accelerations (body frame)/1
  ensure data type is unit16/1 -> convert motor comand to thrust/1(cmd [uint16])
  convert motor comand to thrust/1(thrust [N]) -> Demux/1
  Mux/1 -> per motor thrust [N]/1, Full equations of motions implemented in one shot/1(thrusts [N])
  Demux/4 -> DC motor low pass filter3/1
  DC motor low pass filter3/1 -> Mux/4
  Demux/3 -> DC motor low pass filter2/1
  DC motor low pass filter2/1 -> Mux/3
  Demux/2 -> DC motor low pass filter1/1
  DC motor low pass filter1/1 -> Mux/2
  Demux/1 -> DC motor low pass filter/1
  DC motor low pass filter/1 -> Mux/1

== system Crazyflie_Library/Crazyflie_Model/convert thrust [N] to [uint16] motor commands ==
  note: CONVERT THRUST IN NEWTONS TO MOTOR COMMAND AS uint16 VALUE
      | > This find the positive solution of the equation:
      | thust [N] = nrotor_vehicle_thrust_max * ( cmd_2_newtons_conversion_quadratic_coefficient * cmd^2 + cmd_2_newtons_conversion_linear_coefficient * cmd )
      |
      | > This sub-system acts element-wise on the input, i.e., the output is a vector of the same length as the input
  thrust [N] : Inport
  -b + sqrt(b^2 - 4ac)) : Sum
  Data Type Conversion : DataTypeConversion  OutDataTypeStr=uint16
  Saturation on cmd : Saturate  UpperLimit=param.cmd_max  LowerLimit=param.cmd_min  ZeroCross=off
  b^2 - 4ac : Sum  Inputs=+-
  ensure non-negative : MinMax  Function=max  Inputs=2
  "part of quadratic formula: \"-b\"" : Constant  Value=-param.cmd_2_newtons_conversion_linear_coefficient
  "part of quadratic formula: \"1/(2a)\"" : Gain  Gain=1 / ( 2 * param.cmd_2_newtons_conversion_quadratic_coefficient )
  "part of quadratic formula: \"4ac\"" : Gain  Gain=-(4 * param.cmd_2_newtons_conversion_quadratic_coefficient) ./ param.nrotor_vehicle_thrust_max
  "part of quadratic formula: \"b^2\"" : Constant  Value=param.cmd_2_newtons_conversion_linear_coefficient^2
  sqrt(b^2 - 4ac)) : Sqrt  SaturateOnIntegerOverflow=on
  zero : Constant  Value=0
  cmd [uint16] : Outport
  wires:
  thrust [N]/1 -> "part of quadratic formula: \"4ac\""/1
  Saturation on cmd/1 -> Data Type Conversion/1
  Data Type Conversion/1 -> cmd [uint16]/1
  "part of quadratic formula: \"4ac\""/1 -> b^2 - 4ac/2
  "part of quadratic formula: \"b^2\""/1 -> b^2 - 4ac/1
  b^2 - 4ac/1 -> ensure non-negative/1
  ensure non-negative/1 -> sqrt(b^2 - 4ac))/1
  "part of quadratic formula: \"-b\""/1 -> -b + sqrt(b^2 - 4ac))/1
  sqrt(b^2 - 4ac))/1 -> -b + sqrt(b^2 - 4ac))/2
  -b + sqrt(b^2 - 4ac))/1 -> "part of quadratic formula: \"1/(2a)\""/1
  "part of quadratic formula: \"1/(2a)\""/1 -> Saturation on cmd/1
  zero/1 -> ensure non-negative/2
